simulink model "PD_Simulation"  (Simulink 7.8)
settings: Solver=ode45  StartTime=0.0  StopTime=20  MaxStep=0.01  RelTol=1e-3
values from neighbouring files (symbols this model uses):
  P = zeros(7,1)    [Constants.m]
  X0 = [pi/2+.1 -.05 0 0]    [ABC.m]    (also in Constants.m = [pi/2 -pi 0 0]'; Lab1DemoParam.m = [.05 0 -.02 0])
settings Model: Creator=shahin  LastModifiedBy=salmas5
settings GRTTargetCC: CombineOutputUpdateFcns=on

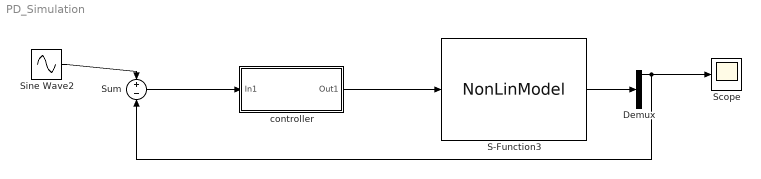
== system PD_Simulation ==
  Demux : Demux
  S-Function3 : S-Function  FunctionName=NonLinModel  Parameters=X0,P  EnableBusSupport=off
  Scope : Scope
      settings: YMin=0.5  YMax=2.7
  Sine Wave2 : Sin  Amplitude=60*(pi/180)  Bias=pi/2  Frequency=(1/3)*(2*pi)  SampleTime=0
  Sum : Sum  Inputs=+-
  controller : Subsystem
  wires:
  Sine Wave2/1 -> Sum/1
  Sum/1 -> controller/1(In1)
  controller/1(Out1) -> S-Function3/1
  S-Function3/1 -> Demux/1
  Demux/1 -> Sum/2, Scope/1

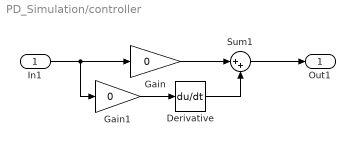
== system PD_Simulation/controller ==
  In1 : Inport
  Derivative : Derivative
  Gain : Gain  Gain=0
  Gain1 : Gain  Gain=0
  Sum1 : Sum  Inputs=|++
  Out1 : Outport
  wires:
  Gain1/1 -> Derivative/1
  In1/1 -> Gain1/1, Gain/1
  Derivative/1 -> Sum1/2
  Gain/1 -> Sum1/1
  Sum1/1 -> Out1/1
